simulink model "RLC"  (R2016b)
settings: Solver=VariableStepAuto  StartTime=0.0  StopTime=4*10^-2  MaxStep=1*10^-6  RelTol=1e-3
undefined symbols (not defined in the file or in its folder): K1, K2, K3
settings Model: Creator=ee105-abq  LastModifiedBy=ee105-abq

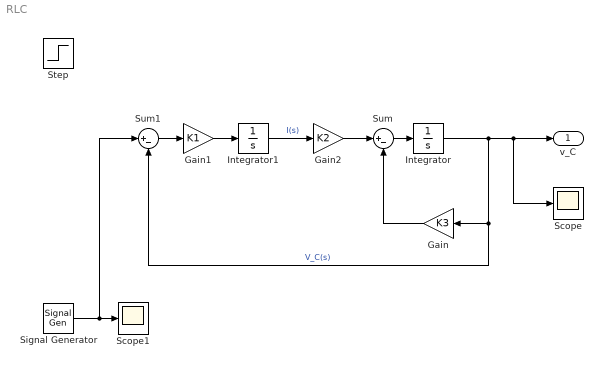
== system RLC ==
  Gain : Gain  Gain=K3
  Gain1 : Gain  Gain=K1
  Gain2 : Gain  Gain=K2
  Integrator : Integrator  InitialCondition=1
  Integrator1 : Integrator
  Scope : Scope
  Scope1 : Scope
  Signal Generator : SignalGenerator  WaveForm=square  Frequency=250
  Step : Step  Time=0  SampleTime=0
  Sum : Sum  Inputs=|+-
  Sum1 : Sum  Inputs=|+-
  "v_C " : Outport
  wires:
  Sum1/1 -> Gain1/1
  Gain1/1 -> Integrator1/1
  Integrator1/1 -> Gain2/1  "I(s)"
  Gain2/1 -> Sum/1
  Sum/1 -> Integrator/1
  Integrator/1 -> Sum1/2, Gain/1, Scope/1, "v_C "/1  "V_C(s)"
  Gain/1 -> Sum/2
  Signal Generator/1 -> Sum1/1, Scope1/1
